simulink model "capitol3pb6"  (R2013a)
settings: Solver=ode45  StartTime=0.0  StopTime=28800  RelTol=1e-3
undefined symbols (not defined in the file): des, gcbh
settings Model: Creator=user  LastModifiedBy=user

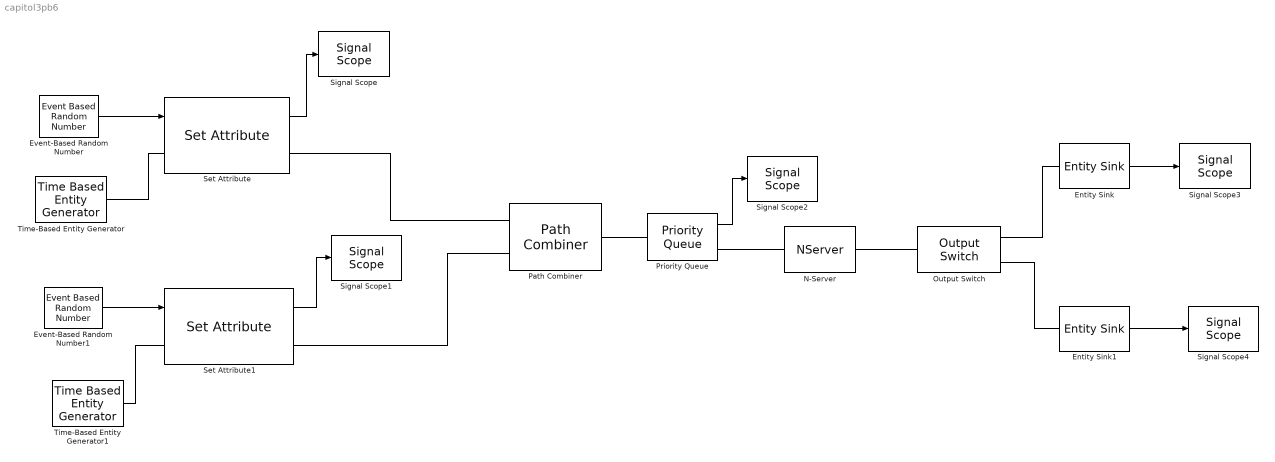
== system capitol3pb6 ==
  Entity Sink : EntitySink  StatNumberArrived=on
  Entity Sink1 : EntitySink  StatNumberArrived=on
  Event-Based Random Number : EventBasedRandomNumber  Distribution=Uniform  minUnif=210  maxUnif=390
  Event-Based Random Number1 : EventBasedRandomNumber  Distribution=Uniform  minUnif=70  maxUnif=130
  N-Server : NServer  NumberOfServers=2  ServiceTimeFrom=Attribute
  Output Switch : OutputSwitch  NumberOutputPorts=2  SwitchingCriterion=From attribute  AttributeName=PriorityAttributeName
  Path Combiner : PathCombiner  NumberInputPorts=2
  Priority Queue : PriorityQueue  StatAverageQueueLength=on
      settings: OutputPortMap=o3
  Set Attribute : SetAttribute  AttributeName=PriorityAttributeName|ServiceTime  AttributeFrom=Dialog|Signal port  AttributeValue=1|1  AttributeTreatAsVector=1|1  StatNumberDeparted=on  EvaluatedAttributeValue={ 1;[]}
      settings: InputPortMap=u1
  Set Attribute1 : SetAttribute  AttributeName=PriorityAttributeName|ServiceTime  AttributeFrom=Dialog|Signal port  AttributeValue=2|1  AttributeTreatAsVector=1|1  StatNumberDeparted=on  EvaluatedAttributeValue={ 2;[]}
      settings: InputPortMap=u1
  Signal Scope{,1..4} (5 alike) : SignalScope  LoadFcn=des.scope.CallbackSupport('seLoadFcn',gcbh)  StartFcn=des.scope.CallbackSupport('seStartFcn',gcbh)  StopFcn=des.scope.CallbackSupport('seStopFcn',gcbh)
      settings: CopyFcn=des.scope.CallbackSupport('seCopyFcn',gcbh)  DeleteFcn=des.scope.CallbackSupport('seDeleteFcn',gcbh)  PreSaveFcn=des.scope.CallbackSupport('sePreSaveFcn',gcbh)  NameChangeFcn=des.scope.CallbackSupport('seNameChangeFcn',gcbh)  OpenFcn=des.scope.CallbackSupport('seOpenFcn',gcbh)
  Time-Based Entity Generator : TimeBasedEntityGenerator  Distribution=Uniform  Minimum=60  Maximum=780  Mean=12
  Time-Based Entity Generator1 : TimeBasedEntityGenerator  Distribution=Uniform  Minimum=120  Maximum=600  Mean=12
  wires:
  Event-Based Random Number/1 -> Set Attribute/1
  Event-Based Random Number1/1 -> Set Attribute1/1
  Set Attribute/1 -> Signal Scope/1
  Set Attribute1/1 -> Signal Scope1/1
  Entity Sink/1 -> Signal Scope3/1
  Entity Sink1/1 -> Signal Scope4/1
  Priority Queue/1 -> Signal Scope2/1
  connections:
  Time-Based Entity Generator/RConn1 -- Set Attribute/LConn1
  Time-Based Entity Generator1/RConn1 -- Set Attribute1/LConn1
  Set Attribute/RConn1 -- Path Combiner/LConn1
  Set Attribute1/RConn1 -- Path Combiner/LConn2
  Path Combiner/RConn1 -- Priority Queue/LConn1
  N-Server/RConn1 -- Output Switch/LConn1
  Output Switch/RConn2 -- Entity Sink1/LConn1
  Output Switch/RConn1 -- Entity Sink/LConn1
  Priority Queue/RConn1 -- N-Server/LConn1
